simulink model "YN_Detector"  (R2020a)
settings: Solver=FixedStepDiscrete  StartTime=0.0  StopTime=1.2  RelTol=1e-3
values from neighbouring files (symbols this model uses):
  InputThreshold = 0.006    [Model_Simulator.m]
  YNThreshold = 0.8    [Model_Simulator.m]
libraries: dspstat3 x4, dspfdesign x2, dspvision x1
settings Model: ParamWorkspaceSource=ReferencedWorkspace  TunableVars=InputThreshold,MaxWindow,SimulationTime,YNThreshold  TunableVarsStorageClass=Auto,ExportedGlobal,Auto,Auto  TunableVarsTypeQualifier=const,,const,const  Creator=jose_  LastModifiedBy=jose_
settings SolverCC: AutoInsertRateTranBlk=on
settings DataIOCC: LimitDataPoints=on  SaveOutput=off  SignalLogging=off  SaveTime=off
settings OptimizationCC: DefaultParameterBehavior=Inlined  UseDivisionForNetSlopeComputation=on  GainParamInheritBuiltInType=on  UseFloatMulNetSlope=on  UseSpecifiedMinMax=on  EnhancedBackFolding=on  CachingGlobalReferences=on  PassReuseOutputArgsAs=Individual arguments  NoFixptDivByZeroProtection=on  EfficientFloat2IntCast=on  LifeSpan=1  OptimizeBlockOrder=speed  DifferentSizesBufferReuse=on  EfficientTunableParamExpr=on
settings DebuggingCC: AlgebraicLoopMsg=error  SingleTaskRateTransMsg=error  ParameterTunabilityLossMsg=error  AllowSymbolicDim=off  SFUnexpectedBacktrackingDiag=warning  SFNoUnconditionalDefaultTransitionDiag=warning  SFExecutionAtInitializationDiag=none  ArithmeticOperatorsInVariantConditions=warning
settings HardwareCC: ProdBitPerPointer=32  ProdBitPerSizeT=32  ProdBitPerPtrDiffT=32  ProdLargestAtomicInteger=Long  ProdLargestAtomicFloat=Double  ProdWordSize=32  ProdLongLongMode=on  ProdHWDeviceType=ARM Compatible->ARM Cortex
settings SFSimCC: SimUseLocalCustomCode=off  MATLABDynamicMemAlloc=off  CustomCodeUndefinedFunction=UseInterfaceOnly
settings RTWCC: SystemTargetFile=ert.tlc  GenCodeOnly=on  TemplateMakefile=ert_default_tmf  GenerateReport=on  RTWUseLocalCustomCode=off  BuildConfiguration=Faster Runs  IncludeHyperlinkInReport=on  LaunchReport=on  GenerateTraceInfo=on  GenerateTraceReport=on  GenerateTraceReportSl=on  GenerateTraceReportSf=on  GenerateTraceReportEml=on  GenerateCodeMetricsReport=on
settings CodeAppCC: ForceParamTrailComments=on  IgnoreCustomStorageClasses=off  OperatorAnnotations=on  SimulinkDataObjDesc=on  SFDataObjDesc=on  CustomSymbolStrGlobalVar=rt$N$M  CustomSymbolStrType=$N$M  CustomSymbolStrFcn=$N$M$F  CustomSymbolStrMacro=$N$M  InsertBlockDesc=on  InternalIdentifier=Classic  InlinedPrmAccess=Macros
settings ERTTargetCC: CodeReplacementLibrary=ARM Cortex-M (CMSIS)  GenerateSampleERTMain=on  IncludeMdlTerminateFcn=off  CombineSignalStateStructs=on  SuppressErrorStatus=on  SupportAbsoluteTime=off  MultiInstanceERTCode=on  CodeInterfacePackaging=Reusable function  SupportNonFinite=off  SupportComplex=off  InlinedParameterPlacement=NonHierarchical  ERTCustomFileTemplate=example_file_process.tlc  ERTFilePackagingFormat=CompactWithDataFile
settings ConfigComp: CovMetricSettings=dw  CovHtmlReporting=on  CovSaveCumulativeToWorkspaceVar=on  CovSaveSingleToWorkspaceVar=on  CovExternalEMLEnable=off  CovSFcnEnable=off

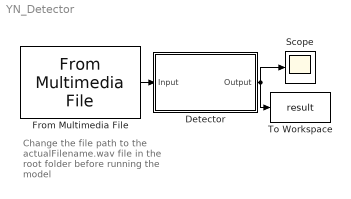
== system YN_Detector ==
  note: Change the file path to the actualFilename.wav file in the root folder before running the model
  Detector : Subsystem
  From Multimedia File : dspvision/From Multimedia File  inputFilename=C:\Users\jose_\OneDrive\Ingenieria\DSP\DSP_LAB_PROJECT\MATLAB\actualFilename.wav  readRange=[1 Inf]  loop=on  numPlays=1  outputStreams=Audio only  videoDataType=single  audioDataType=double  inheritSampleTime=on  userDefinedSampleTime=1/30  noAudioOutput=off  isIntensityVideo=off  fourcc=RGB  colorVideoFormat=Separate color signals  outputEOF=off  dataOrg=Column-major  audioFrameSize=DMA_BlockSize  computeAudioFrameSize=off  outSamplingMode=Sample based
  Scope : Scope
  To Workspace : ToWorkspace  VariableName=result  SampleTime=-1
      settings: MaxDataPoints=1  Save2DSignal=2-D array (concatenate along first dimension)
  wires:
  From Multimedia File/1 -> Detector/1(Input)
  Detector/1(Output) -> Scope/1, To Workspace/1

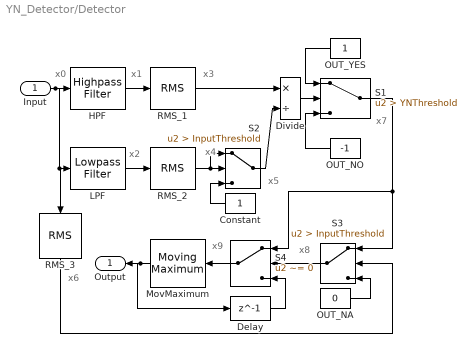
== system YN_Detector/Detector ==
  note: x8
  note: x5
  note: x1
  note: x2
  note: x9
  note: x0
  note: x4
  note: x7
  note: x6
  note: x3
  Input : Inport  PortDimensions=128
  Constant : Constant
  Delay : Delay  DelayLength=1  StateName=u
  Divide : Product  Inputs=*/
  HPF : dspfdesign/Highpass Filter  FilterType=FIR  DesignForMinimumOrder=on  FilterOrder=50  StopbandFrequency=HPF.sb  PassbandFrequency=HPF.pb  StopbandAttenuation=80  PassbandRipple=0.1  InheritSampleRate=off  SampleRate=Fs_system  SimulateUsing=Interpreted execution  roundingMode=Simplest  coeffsDataTypeStr=fixdt(1,16)
  LPF : dspfdesign/Lowpass Filter  FilterType=FIR  DesignForMinimumOrder=on  FilterOrder=50  PassbandFrequency=LPF.pb  StopbandFrequency=LPF.sb  PassbandRipple=0.1  StopbandAttenuation=80  InheritSampleRate=off  SampleRate=Fs_system  SimulateUsing=Interpreted execution  roundingMode=Simplest  coeffsDataTypeStr=fixdt(1,16)
  MovMaximum : dspstat3/Moving Maximum  SpecifyWindowLength=on  WindowLength=MaxWindow  SimulateUsing=Interpreted execution
      settings: SourceProductBaseCode=DS
  OUT_NA : Constant  Value=0
  OUT_NO : Constant  Value=-1
  OUT_YES : Constant
  RMS_1 : dspstat3/RMS  run=off  directionMode=Each column  dimension=1  InputProcessing=Columns as channels (frame based)  reset_popup=None
  RMS_2 : dspstat3/RMS  run=off  directionMode=Each column  dimension=1  InputProcessing=Columns as channels (frame based)  reset_popup=None
  RMS_3 : dspstat3/RMS  run=off  directionMode=Each column  dimension=1  InputProcessing=Columns as channels (frame based)  reset_popup=None
  S1 : Switch  Criteria=u2 > Threshold  Threshold=YNThreshold
  S2 : Switch  Criteria=u2 > Threshold  Threshold=InputThreshold
  "S3 " : Switch  Criteria=u2 > Threshold  Threshold=InputThreshold
  S4 : Switch  Criteria=u2 ~= 0  Threshold=0.012
  Output : Outport
  wires:
  Input/1 -> RMS_3/1, LPF/1, HPF/1
  OUT_YES/1 -> S1/1
  RMS_2/1 -> S2/1, S2/2
  Constant/1 -> S2/3
  MovMaximum/1 -> Delay/1, Output/1
  S1/1 -> "S3 "/1, S4/1
  S2/1 -> Divide/2
  RMS_3/1 -> "S3 "/2
  Divide/1 -> S1/2
  RMS_1/1 -> Divide/1
  HPF/1 -> RMS_1/1
  LPF/1 -> RMS_2/1
  OUT_NA/1 -> "S3 "/3
  "S3 "/1 -> S4/2
  Delay/1 -> S4/3
  OUT_NO/1 -> S1/3
  S4/1 -> MovMaximum/1
